simulink model "ZynqBF_2tx_tb"  (R2018b)
settings: Solver=FixedStepAuto  StartTime=0.0  StopTime=5e5  FixedStep=1  RelTol=1e-3
settings Model: SimulationMode=accelerator  PauseTimes=20000  Creator=jason  LastModifiedBy=jason

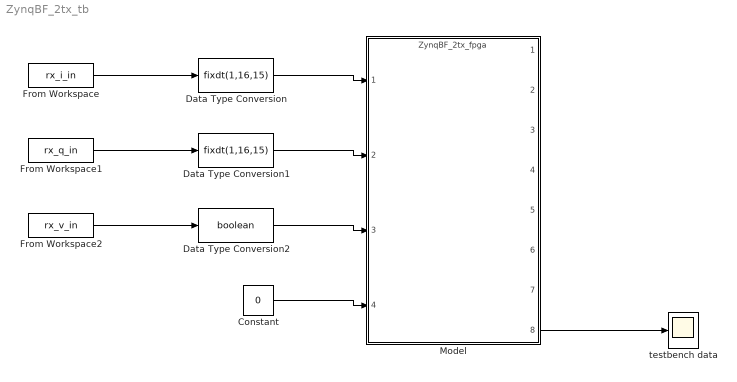
== system ZynqBF_2tx_tb ==
  Constant : Constant  Value=0  OutDataTypeStr=uint16  SampleTime=-1
  Data Type Conversion : DataTypeConversion  OutDataTypeStr=fixdt(1,16,15)
  Data Type Conversion1 : DataTypeConversion  OutDataTypeStr=fixdt(1,16,15)
  Data Type Conversion2 : DataTypeConversion  OutDataTypeStr=boolean
  From Workspace : FromWorkspace  VariableName=rx_i_in  SampleTime=0  OutputAfterFinalValue=Holding final value
  From Workspace1 : FromWorkspace  VariableName=rx_q_in  SampleTime=0  OutputAfterFinalValue=Holding final value
  From Workspace2 : FromWorkspace  VariableName=rx_v_in  SampleTime=0  OutputAfterFinalValue=Setting to zero
  Model : ModelReference  ModelNameDialog=ZynqBF_2tx_fpga  SimulationMode=Normal  ModelReferenceVersion=1.667
  testbench data : Scope
  wires:
  From Workspace/1 -> Data Type Conversion/1
  From Workspace2/1 -> Data Type Conversion2/1
  From Workspace1/1 -> Data Type Conversion1/1
  Data Type Conversion/1 -> Model/1
  Data Type Conversion1/1 -> Model/2
  Data Type Conversion2/1 -> Model/3
  Constant/1 -> Model/4
  Model/8 -> testbench data/1
